simulink model "PWMrectifier"  (R2024a)
settings: Solver=ode15s  StartTime=0.0  StopTime=5  MaxStep=1e-5  RelTol=1e-4  AbsTol=1e-6
libraries: spsIGBTDiodeLib x4, spsSeriesRLCBranchLib x3, spsVoltageMeasurementLib x2, spsACVoltageSourceLib x1, spsCurrentMeasurementLib x1, spsSecondOrderFilterLib x1, powerlib_extras x1, sps_lib x1
settings Model: Creator=SAI DEEPAK  LastModifiedBy=SAI DEEPAK
settings SolverCC: ZeroCrossControl=EnableAll
settings DataIOCC: ReturnWorkspaceOutputs=off

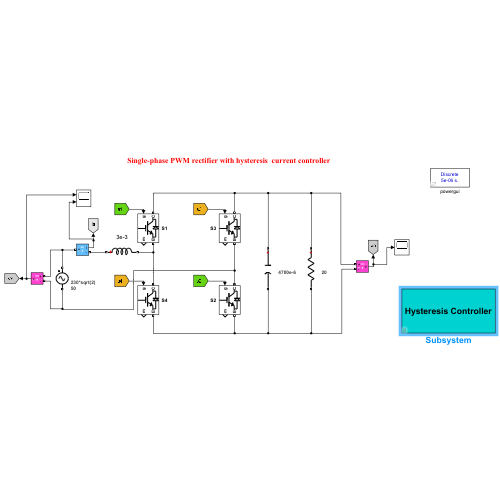
[thumbnail: Simulink's stored preview of the top-level diagram]
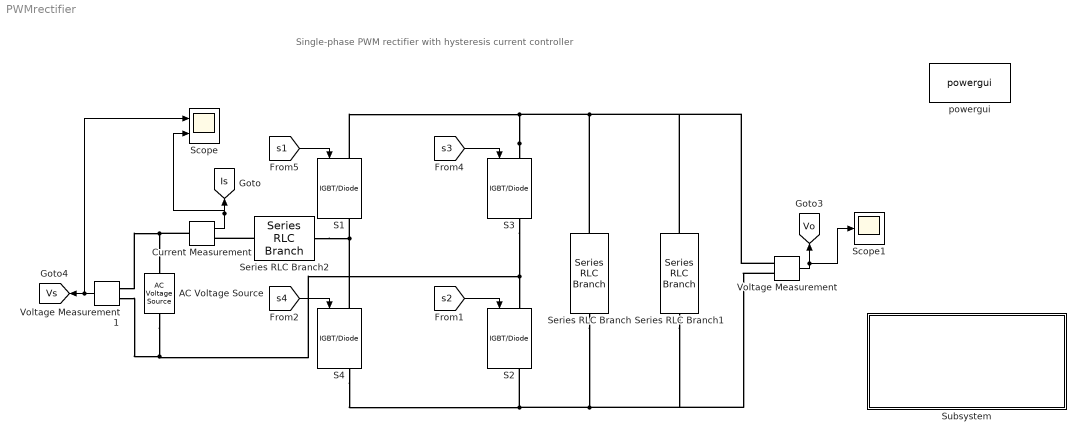
== system PWMrectifier ==
  note: Single-phase PWM rectifier with hysteresis current controller
  AC Voltage Source : spsACVoltageSourceLib/AC Voltage Source  Amplitude=230*sqrt(2)  Phase=0  Frequency=50  SampleTime=0  Measurements=None  BusType=swing  Pref=10e3  Qref=0  Qmin=-inf  Qmax=+inf
      settings: AttributesFormatString=|
      | %<Amplitude>
      | %<Frequency>
  Current Measurement : spsCurrentMeasurementLib/Current Measurement  PhasorSimulation=off  OutputType=Complex  PSBequivalent=0
  S{1..4} (4 alike) : spsIGBTDiodeLib/IGBT//Diode  Ron=1e-3  Rs=1e5  Cs=inf  Measurements=on
  Scope : Scope  NumInputPorts=2
  Scope1 : Scope
  Series RLC Branch : spsSeriesRLCBranchLib/Series RLC Branch  LConnTagsString=__new0  RConnTagsString=__new0  BranchType=C  Resistance=1  Inductance=1e-3  SetiL0=off  InitialCurrent=0  Capacitance=4700e-6  Setx0=off  InitialVoltage=0  Measurements=None
      settings: AttributesFormatString=%<Capacitance>
  Series RLC Branch1 : spsSeriesRLCBranchLib/Series RLC Branch  LConnTagsString=__new0  RConnTagsString=__new0  BranchType=R  Resistance=20  Inductance=1e-3  SetiL0=off  InitialCurrent=0  Capacitance=1e-6  Setx0=off  InitialVoltage=0  Measurements=None
      settings: AttributesFormatString=%<Resistance>
  Series RLC Branch2 : spsSeriesRLCBranchLib/Series RLC Branch  LConnTagsString=__new0  RConnTagsString=__new0  BranchType=L  Resistance=1  Inductance=3e-3  SetiL0=off  InitialCurrent=0  Capacitance=1e-6  Setx0=off  InitialVoltage=0  Measurements=None
      settings: AttributesFormatString=%<Inductance>
  Subsystem : Subsystem  mask{InputProcessing=Elements as channels (sample based), LockScale=off, OffOutputValue=0, OffSwitchValue=-0.5, OnOutputValue=1, OnSwitchValue=0.5, OutDataTypeStr=Inherit: All ports same datatype, OutMax=[], OutMin=[], SampleTime=-1, ZeroCross=on}
      mask prompts: InputProcessing "Simulink:blkprm_prompts:InputProcessing"; LockScale "Simulink:blkprm_prompts:LockScale"; OffOutputValue "Simulink:blkprm_prompts:RelayOutputWhenOff"; OffSwitchValue "Simulink:blkprm_prompts:RelaySwitchOffPoint"; OnOutputValue "Simulink:blkprm_prompts:RelayOutputWhenOn"; OnSwitchValue "Simulink:blkprm_prompts:RelaySwitchOnPoint"; OutDataTypeStr "Simulink:blkprm_prompts:OUTPUT_UNIFIEDDATATYPE"; OutMax "Simulink:blkprm_prompts:OutputDesignMax"; OutMin "Simulink:blkprm_prompts:OutputDesignMin"; SampleTime "Simulink:blkprm_prompts:AllBlksSampleTime"; ZeroCross "Simulink:blkprm_prompts:AllBlksEnableZC"
      mask TypeOptions InputProcessing: Relay(hysteresis)/InputProcessing
      mask TypeOptions LockScale: Relay(hysteresis)/LockScale
      mask TypeOptions OffOutputValue: Relay(hysteresis)/OffOutputValue
      mask TypeOptions OffSwitchValue: Relay(hysteresis)/OffSwitchValue
      mask TypeOptions OnOutputValue: Relay(hysteresis)/OnOutputValue
      mask TypeOptions OnSwitchValue: Relay(hysteresis)/OnSwitchValue
      mask TypeOptions OutDataTypeStr: Relay(hysteresis)/OutDataTypeStr
      mask TypeOptions OutMax: Relay(hysteresis)/OutMax
      mask TypeOptions OutMin: Relay(hysteresis)/OutMin
      mask TypeOptions SampleTime: Relay(hysteresis)/SampleTime
      mask TypeOptions ZeroCross: Relay(hysteresis)/ZeroCross
      mask DialogControl InputProcessing Prompt: Input processing:
      mask DialogControl LockScale Prompt: Lock output data type setting against changes by the fixed-point tools
      mask DialogControl OffOutputValue Prompt: Output when off:
      mask DialogControl OffSwitchValue Prompt: Switch off point:
      mask DialogControl OnOutputValue Prompt: Output when on:
      mask DialogControl OnSwitchValue Prompt: Switch on point:
      mask DialogControl OutDataTypeStr Prompt: Output data type:
      mask DialogControl OutMax Prompt: Output maximum:
      mask DialogControl OutMin Prompt: Output minimum:
      mask DialogControl SampleTime Prompt: Sample time (-1 for inherited):
      mask DialogControl ZeroCross Prompt: Enable zero-crossing detection
      mask Display: disp('Hysteresis Controller');
  Voltage Measurement : spsVoltageMeasurementLib/Voltage Measurement  PhasorSimulation=off  OutputType=Complex  PSBequivalent=0
  Voltage Measurement1 : spsVoltageMeasurementLib/Voltage Measurement  PhasorSimulation=off  OutputType=Complex  PSBequivalent=0
  powergui : sps_lib/powergui  Priority=1  SimulationMode=Discrete  SampleTime=5e-6  frequency=60  Iterations=50  frequencyindice=50  Pbase=100e6  ErrMax=1e-4  UnitsV=kV  UnitsW=MW  buscounter=0  FunctionMessages=off  echomessages=off  EnableUseOfTLC=off  CurrentSourceSwitches=off  DisableSnubberDevices=off  DisableRonSwitches=off  DisableVfSwitches=off  DisplayEquations=off  AutomaticDiscreteSolvers=off  SolverType=Tustin/Backward Euler (TBE)  Interpol=off  ExternalGateDelay=off  methode=off  Ts=100  x0status=blocks  SPID=on  SwTol=0  HookPort=off  NonlinearTolerance=1e-4  nMaxIteration=100  ContinueOnMaxIteration=off  RestoreLinks=warning  ResistiveCurrentMeasurement=off  Frange=[0:2:500]  Ylog=off  Xlog=on  ShowGrid=off  save=off  variable=ZData  structure=0  ZoomFFT=off  StartTime=0.0  cycles=1  DisplayStyle=1  fundamental=60  FreqAxis=off  MaxFrequency=1000  frequencyindicesteady=1  RmsSteady=1  display=off
  tag scope: Is=global, Vo=global, Vs=global
  wires:
  [s2] -> S2/1
  [s4] -> S4/1
  Current Measurement/1 -> Scope/2, [Is]
  [s3] -> S3/1
  Voltage Measurement/1 -> Scope1/1, [Vo]
  Voltage Measurement1/1 -> Scope/1, [Vs]
  [s1] -> S1/1
  connections:
  S4/RConn1 -- Voltage Measurement/LConn2 -- Series RLC Branch1/RConn1 -- Series RLC Branch/RConn1 -- S2/RConn1
  AC Voltage Source/LConn1 -- Voltage Measurement1/LConn2 -- S3/RConn1 -- S2/LConn1
  Series RLC Branch2/RConn1 -- S4/LConn1 -- S1/RConn1
  Current Measurement/LConn1 -- Voltage Measurement1/LConn1 -- AC Voltage Source/RConn1
  S3/LConn1 -- S1/LConn1 -- Voltage Measurement/LConn1 -- Series RLC Branch1/LConn1 -- Series RLC Branch/LConn1
  Series RLC Branch2/LConn1 -- Current Measurement/RConn1

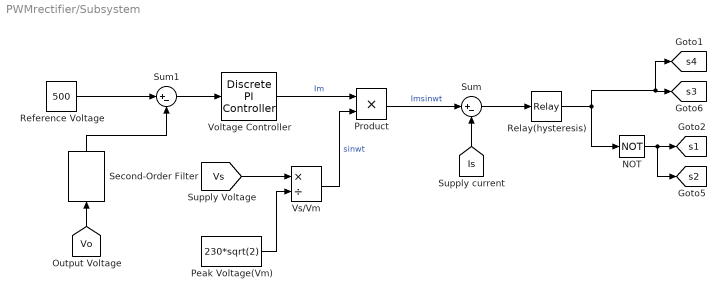
== system PWMrectifier/Subsystem ==
  NOT : Logic  Operator=NOT  IconShape=distinctive  AllPortsSameDT=off  OutDataTypeStr=boolean
  Peak Voltage(Vm) : Constant  Value=230*sqrt(2)  SampleTime=-1
  Product : Product
  Reference Voltage : Constant  Value=500  SampleTime=-1
  Relay(hysteresis) : Relay  OnSwitchValue=OnSwitchValue  OffSwitchValue=OffSwitchValue  OnOutputValue=OnOutputValue  OffOutputValue=OffOutputValue  OutMin=OutMin  OutMax=OutMax  SampleTime=SampleTime
  Second-Order Filter : spsSecondOrderFilterLib/Second-Order Filter  FilterType=Bandstop (Notch)  Fo=100  Zeta=1  Ts=0  Initialize=off  Vac_Init="[0,  0,  60]"  Vdc_Init=0  PlotResponse=off  FreqRange=[0, 500, 1]
      settings: LibrarySourceBlock=|
      | sps_lib/Control/Filters/Second-Order
      | Filter
  Sum : Sum  Inputs=|+-
  Sum1 : Sum  Inputs=|+-
  Voltage Controller : powerlib_extras/Discrete  Control Blocks/Discrete PI Controller  Kp=2  Ki=5  Par_Limits=[1e6 -1e6]  Init=0  Ts=5e-6
  Vs/Vm : Product  Inputs=*/  RndMeth=Zero  SaturateOnIntegerOverflow=on
  tag scope: s1=global, s2=global, s3=global, s4=global
  wires:
  [Is] -> Sum/2
  Vs/Vm/1 -> Product/2  "sinwt"
  Peak Voltage(Vm)/1 -> Vs/Vm/2
  [Vo] -> Second-Order Filter/1
  [Vs] -> Vs/Vm/1
  Sum1/1 -> Voltage Controller/1
  Voltage Controller/1 -> Product/1  "Im"
  Reference Voltage/1 -> Sum1/1
  Sum/1 -> Relay(hysteresis)/1
  Relay(hysteresis)/1 -> NOT/1, [s4], [s3]
  Product/1 -> Sum/1  "Imsinwt"
  NOT/1 -> [s2], [s1]
  Second-Order Filter/1 -> Sum1/2
